simulink model "Problem5_48_BlockDiagram"  (R2020b)
settings: Solver=VariableStepAuto  StartTime=0.0  StopTime=20  RelTol=1e-3
values from neighbouring files (symbols this model uses):
  a = 0.05    [Problem5_48.m]
  e = 0.5    [Problem5_48.m]
  m = 0.2    [Problem5_48.m]
  r = 1.0    (= 1)    [Problem5_48.m]
  x_1_init = 0    [Problem5_27.m]    (also in Problem5_48.m = 9)
  x_2_init = 0    [Problem5_27.m]    (also in Problem5_48.m = 1)
settings Model: Creator=jonathanmoran  LastModifiedBy=jonathanmoran

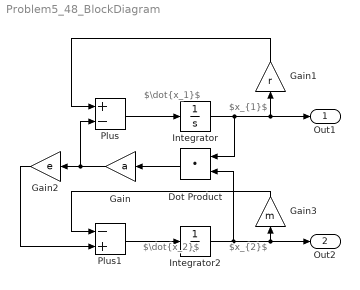
== system Problem5_48_BlockDiagram ==
  note: $\dot{x_1}$
  note: $x_{1}$
  note: $\dot{x_2}$
  note: $x_{2}$
  Dot Product : DotProduct  InputSameDT=on  OutDataTypeStr=Inherit: Inherit via internal rule
  Gain : Gain  Gain=a
  Gain1 : Gain  Gain=r
  Gain2 : Gain  Gain=e
  Gain3 : Gain  Gain=m
  Integrator : Integrator  InitialCondition=x_1_init
  Integrator2 : Integrator  InitialCondition=x_2_init
  Plus : Sum  Inputs=+-
  Plus1 : Sum  Inputs=-+
  Out1 : Outport  SignalName=x_1
  Out2 : Outport  Port=2  SignalName=x_2
  wires:
  Plus/1 -> Integrator/1
  Gain1/1 -> Plus/1
  Gain/1 -> Plus/2, Gain2/1
  Gain3/1 -> Plus1/1
  Plus1/1 -> Integrator2/1
  Dot Product/1 -> Gain/1
  Gain2/1 -> Plus1/2
  Integrator/1 -> Gain1/1, Out1/1, Dot Product/1
  Integrator2/1 -> Dot Product/2, Gain3/1, Out2/1
